simulink model "DifferentialEquations2"  (R2017b)
settings: Solver=VariableStepAuto  StartTime=0.0  StopTime=50.0  RelTol=1e-3
settings Model: Creator=Mahe  LastModifiedBy=Mahe

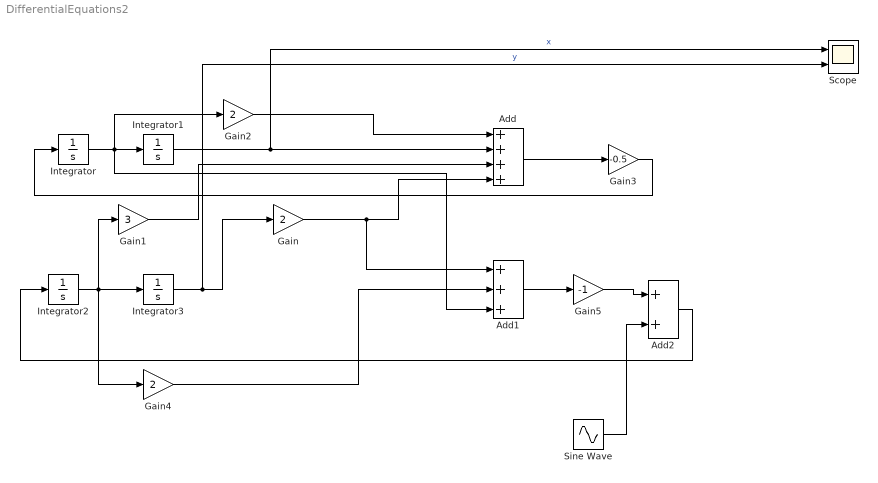
== system DifferentialEquations2 ==
  Add : Sum  Inputs=++++
  Add1 : Sum  Inputs=+++
  Add2 : Sum
  Gain : Gain  Gain=2
  Gain1 : Gain  Gain=3
  Gain2 : Gain  Gain=2
  Gain3 : Gain  Gain=-0.5
  Gain4 : Gain  Gain=2
  Gain5 : Gain  Gain=-1
  Integrator : Integrator
  Integrator1 : Integrator
  Integrator2 : Integrator  InitialCondition=-1
  Integrator3 : Integrator  InitialCondition=1
  Scope : Scope  NumInputPorts=2
  Sine Wave : Sin  Frequency=3.14  SampleTime=0
  wires:
  Integrator2/1 -> Gain4/1, Gain1/1, Integrator3/1
  Integrator/1 -> Add1/3, Gain2/1, Integrator1/1
  Integrator1/1 -> Scope/1, Add/2  "x"
  Integrator3/1 -> Scope/2, Gain/1  "y"
  Gain/1 -> Add1/1, Add/4
  Gain1/1 -> Add/3
  Gain2/1 -> Add/1
  Add/1 -> Gain3/1
  Gain3/1 -> Integrator/1
  Gain4/1 -> Add1/2
  Add1/1 -> Gain5/1
  Gain5/1 -> Add2/1
  Add2/1 -> Integrator2/1
  Sine Wave/1 -> Add2/2
